simulink model "Digital_Twin_Gruppe_1"  (R2024b)
settings: Solver=VariableStepAuto  StartTime=0.0  StopTime=10.0  RelTol=1e-3
settings Model: Creator=justi  LastModifiedBy=justi

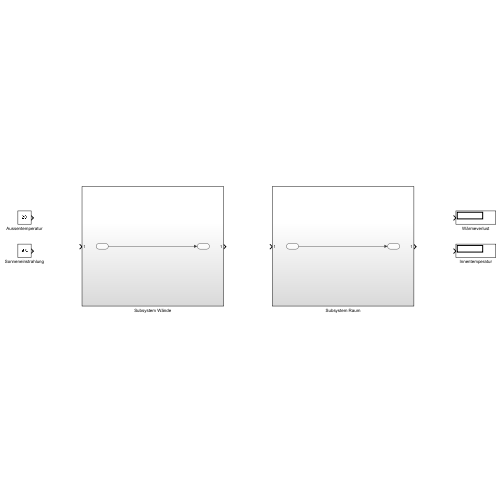
[thumbnail: Simulink's stored preview of the top-level diagram]
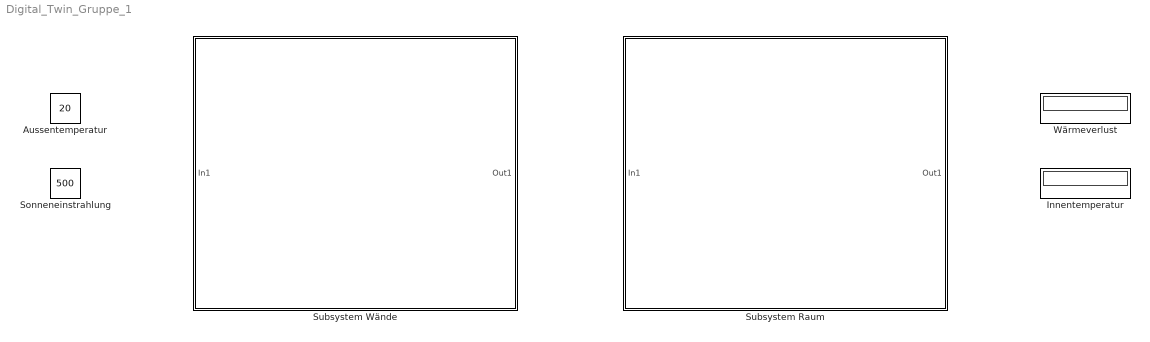
== system Digital_Twin_Gruppe_1 ==
  Aussentemperatur : Constant  Value=20
  Innentemperatur : Display
  Sonneneinstrahlung : Constant  Value=500
  Subsystem Raum : Subsystem
  Subsystem Wände : Subsystem
  Wärmeverlust : Display

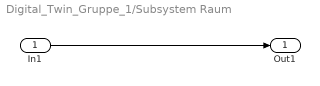
== system Digital_Twin_Gruppe_1/Subsystem Raum ==
  In1 : Inport
  Out1 : Outport
  wires:
  In1/1 -> Out1/1

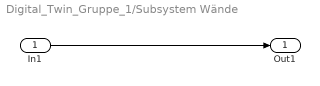
== system Digital_Twin_Gruppe_1/Subsystem Wände ==
  In1 : Inport
  Out1 : Outport
  wires:
  In1/1 -> Out1/1
